simulink model "theta_project"  (R2021a)
settings: Solver=VariableStepAuto  StartTime=0.0  StopTime=25  MaxStep=1e-3  RelTol=1e-3
values from neighbouring files (symbols this model uses):
  g = -9.81    [project.m]
  L = Value_length(i)    [project.m]
  theta_0 = 40    [project.m]
settings Model: Creator=HP  LastModifiedBy=HP

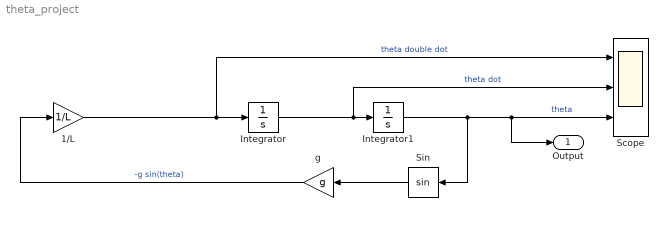
== system theta_project ==
  1/L : Gain  Gain=1/L
  Integrator : Integrator
  Integrator1 : Integrator  InitialCondition=theta_0
  Scope : Scope  NumInputPorts=3
  Sin : Trigonometry
  g : Gain  Gain=g
  Output : Outport
  wires:
  Integrator/1 -> Scope/2, Integrator1/1  "theta dot"
  1/L/1 -> Scope/1, Integrator/1  "theta double dot"
  Integrator1/1 -> Output/1, Scope/3, Sin/1  "theta"
  Sin/1 -> g/1
  g/1 -> 1/L/1  "-g sin(theta)"
